simulink model "task_1"  (R2021b)
settings: Solver=VariableStepAuto  StartTime=0.0  StopTime=0.2  MaxStep=1e-2  RelTol=1e-3
values from neighbouring files (symbols this model uses):
  A = [0 1; a1 a2]    [env_practice_2.m]
  a1 = -4    [env_practice_2.m]
  a2 = -1.6    [env_practice_2.m]
  am1 = -100/9    (= -11.1111111111)    [env_practice_2.m]
  am2 = -50/9    (= -5.55555555556)    [env_practice_2.m]
  B = [0;b]    [env_practice_2.m]
  b = 8    [env_practice_2.m]
  bm = 300/9    (= 33.3333333333)    [env_practice_2.m]
  gb = gb*100    (= 100)    [env_practice_2.m]
  P = [1.34 0.045; 0.045 0.0981]    [env_practice_2.m]
undefined symbols (not defined in the file or in its folder): au, bu, C, ga1, ga2, Gamma
settings Model: Creator=79159  LastModifiedBy=79159
settings SolverCC: ZeroCrossAlgorithm=Adaptive
settings DebuggingCC: IgnoredZcDiagnostic=none

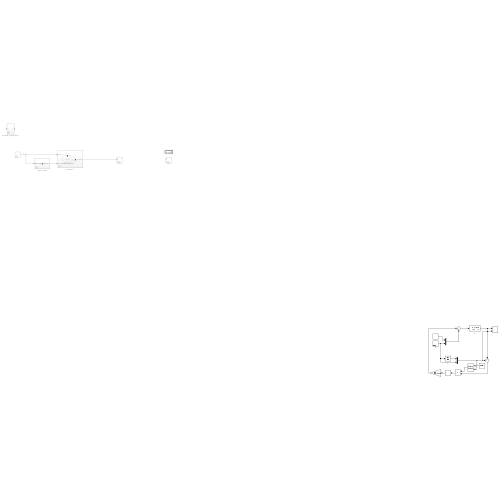
[thumbnail: Simulink's stored preview of the top-level diagram]
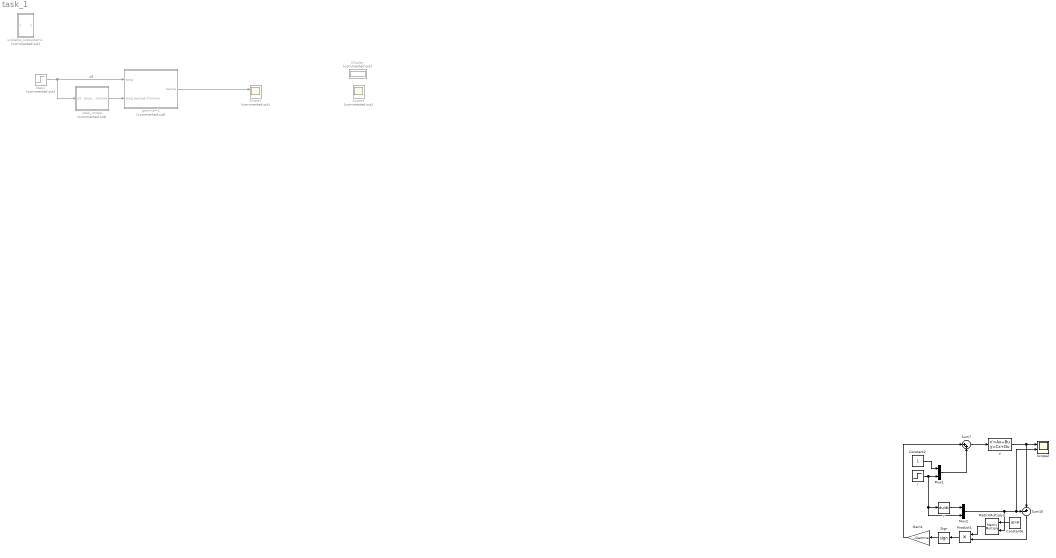
== system task_1 ==
  Constant2 : Constant
  Constant6 : Constant  Value=B'*P  VectorParams1D=off
  Display : Display  Commented=on
      settings: Decimation=2
  Gain4 : Gain  Gain=-Gamma
  MatrixMultiply3 : Product  Multiplication=Matrix(*)
  Mux1 : Mux  Inputs=2
  Mux2 : Mux  Inputs=2
  Product1 : Product
  Scope1 : Scope  Commented=on  NumInputPorts=2
  Scope2 : Scope  NumInputPorts=2
  Scope3 : Scope  Commented=on  NumInputPorts=2
  Sign : Signum
  Step1 : Step  Commented=on  Time=0  SampleTime=0
  Sum10 : Sum  Inputs=-+|
  Sum7 : Sum  Inputs=|++
  gamma=1 : Subsystem  Commented=on
  ideal_model : Subsystem  Commented=on
  r : Step  Time=0.05  SampleTime=0
  r' : Derivative
  unstable_subsystem1 : Subsystem  Commented=on
  y : StateSpace  A=A  B=B  C=C  D=zeros(2)  InitialCondition=0
  wires:
  Step1/1 -> ideal_model/1(u0), gamma=1/1(вход)  "u0"
  ideal_model/1(вход выхода эталона) -> gamma=1/2(вход выхода эталона)
  gamma=1/1(выход) -> Scope1/1
  y/1 -> Sum10/2, Scope2/1
  Sum7/1 -> y/1
  r/1 -> r'/1, Mux2/2, Mux1/2
  Constant2/1 -> Mux1/1
  Mux1/1 -> Sum7/2
  r'/1 -> Mux2/1
  Mux2/1 -> Scope2/2, Sum10/1, MatrixMultiply3/2
  Sum10/1 -> Product1/2
  Sign/1 -> Gain4/1
  Gain4/1 -> Sum7/1
  Product1/1 -> Sign/1
  MatrixMultiply3/1 -> Product1/1
  Constant6/1 -> MatrixMultiply3/1

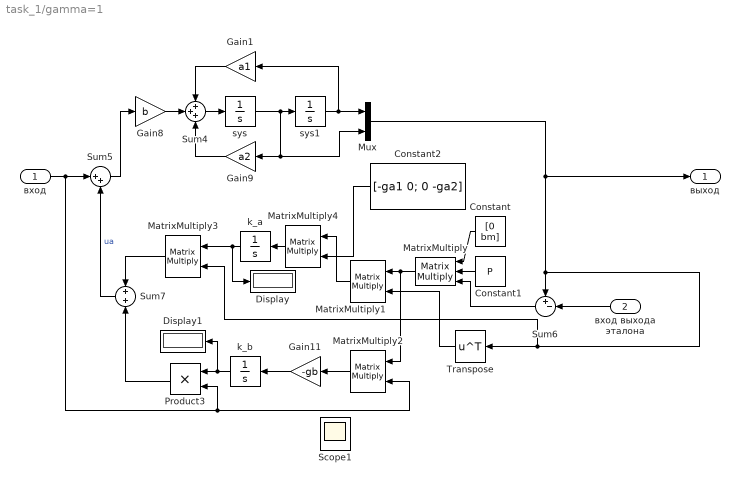
== system task_1/gamma=1 ==
  вход : Inport
  вход выхода эталона : Inport  Port=2
  Constant : Constant  Value=[0 bm]
  Constant1 : Constant  Value=P
  Constant2 : Constant  Value=[-ga1 0; 0 -ga2]
  Display : Display
      settings: Decimation=2
  Display1 : Display
      settings: Decimation=2
  Gain1 : Gain  Gain=a1
  Gain11 : Gain  Gain=-gb
  Gain8 : Gain  Gain=b
  Gain9 : Gain  Gain=a2
  MatrixMultiply : Product  Inputs=3  Multiplication=Matrix(*)
  MatrixMultiply{1..4} (4 alike) : Product  Multiplication=Matrix(*)
  Mux : Mux  Inputs=2
  Product3 : Product
  Scope1 : Scope  NumInputPorts=2
  Sum4 : Sum  Inputs=+++
  Sum5 : Sum  Inputs=|++
  Sum6 : Sum  Inputs=+-|
  Sum7 : Sum
  Transpose : Math  Operator=transpose  SaturateOnIntegerOverflow=on
  k_a : Integrator
  k_b : Integrator
  sys : Integrator
  sys1 : Integrator
  выход : Outport
  wires:
  Product3/1 -> Sum7/2
  k_b/1 -> Display1/1, Product3/1
  Sum7/1 -> Sum5/2  "ua"
  вход/1 -> MatrixMultiply2/2, Product3/2, Sum5/1
  Mux/1 -> MatrixMultiply3/2, Transpose/1, Sum6/1, выход/1
  Constant/1 -> MatrixMultiply/1
  MatrixMultiply2/1 -> Gain11/1
  MatrixMultiply3/1 -> Sum7/1
  Gain11/1 -> k_b/1
  MatrixMultiply/1 -> MatrixMultiply2/1, MatrixMultiply1/1
  вход выхода эталона/1 -> Sum6/2
  Constant1/1 -> MatrixMultiply/2
  Sum6/1 -> MatrixMultiply/3
  Transpose/1 -> MatrixMultiply1/2
  k_a/1 -> MatrixMultiply3/1, Display/1
  MatrixMultiply4/1 -> k_a/1
  MatrixMultiply1/1 -> MatrixMultiply4/1
  Constant2/1 -> MatrixMultiply4/2
  sys1/1 -> Mux/1, Gain1/1
  Sum4/1 -> sys/1
  Gain8/1 -> Sum4/2
  Gain9/1 -> Sum4/3
  sys/1 -> Mux/2, Gain9/1, sys1/1
  Sum5/1 -> Gain8/1
  Gain1/1 -> Sum4/1

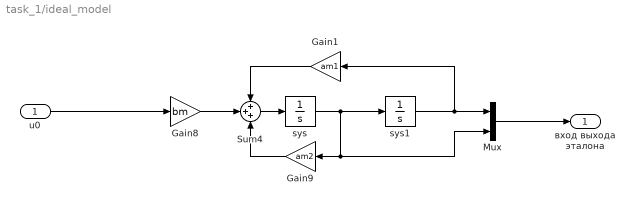
== system task_1/ideal_model ==
  u0 : Inport
  Gain1 : Gain  Gain=am1
  Gain8 : Gain  Gain=bm
  Gain9 : Gain  Gain=am2
  Mux : Mux  Inputs=2
  Sum4 : Sum  Inputs=+++
  sys : Integrator
  sys1 : Integrator
  вход выхода эталона : Outport
  wires:
  Mux/1 -> вход выхода эталона/1
  Gain9/1 -> Sum4/3
  Gain8/1 -> Sum4/2
  Sum4/1 -> sys/1
  sys/1 -> sys1/1, Gain9/1, Mux/2
  u0/1 -> Gain8/1
  sys1/1 -> Gain1/1, Mux/1
  Gain1/1 -> Sum4/1

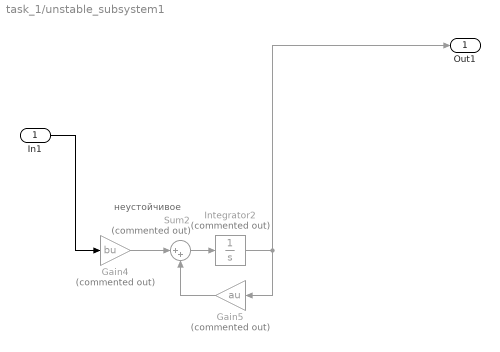
== system task_1/unstable_subsystem1 ==
  note: неустойчивое
  In1 : Inport
  Gain4 : Gain  Commented=on  Gain=bu
  Gain5 : Gain  Commented=on  Gain=au
  Integrator2 : Integrator  Commented=on
  Sum2 : Sum  Commented=on  Inputs=|++
  Out1 : Outport
  wires:
  Gain4/1 -> Sum2/1
  Sum2/1 -> Integrator2/1
  In1/1 -> Gain4/1
  Gain5/1 -> Sum2/2
  Integrator2/1 -> Gain5/1, Out1/1
